simulink model "SetpointTransitionHandler"  (R2016b)
settings: Solver=FixedStepAuto  StartTime=0.0  StopTime=10.0  RelTol=1e-3  EnableMultiTasking=on
settings Model: Creator=march  LastModifiedBy=march
settings SolverCC: EnableConcurrentExecution=on
settings DataIOCC: SaveFormat=StructureWithTime
settings OptimizationCC: BlockReduction=off  OptimizeBlockIOStorage=off  BufferReuse=off  GlobalBufferReuse=off  ExpressionFolding=off  LocalBlockOutputs=off
settings HardwareCC: ProdBitPerPointer=32  ProdBitPerSizeT=32  ProdBitPerPtrDiffT=32  ProdLargestAtomicFloat=None  ProdWordSize=32  ProdLongLongMode=on  ProdHWDeviceType=Generic->32-bit x86 compatible
settings RTWCC: SystemTargetFile=slrt.tlc  TemplateMakefile=slrt_default_tmf  Description=Simulink Real-Time  RTWCompilerOptimization=on

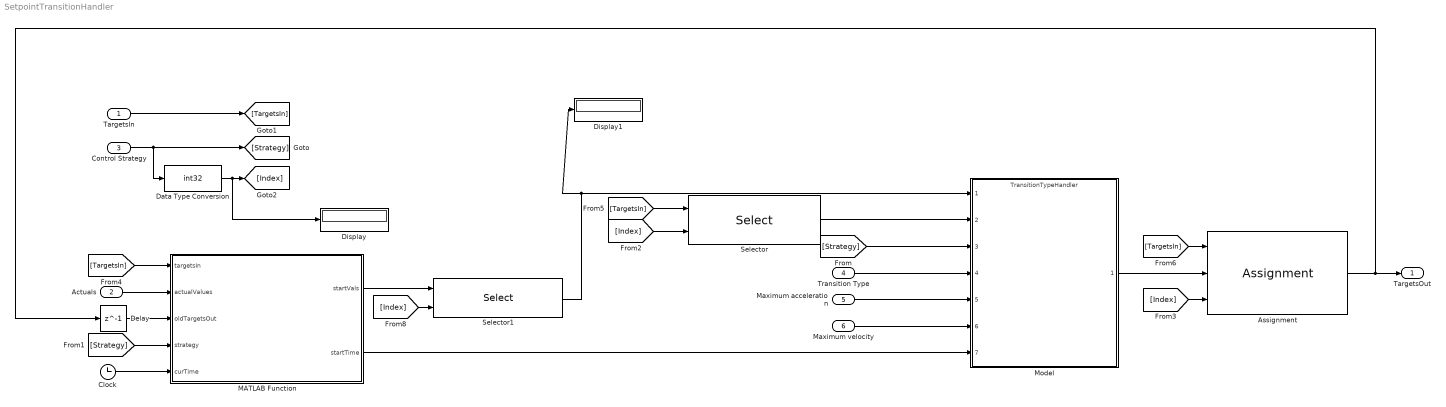
== system SetpointTransitionHandler ==
  TargetsIn : Inport  PortDimensions=[ 3 1 ]
  Actuals : Inport  Port=2  PortDimensions=[ 3 1 ]
  Control Strategy : Inport  Port=3  OutDataTypeStr=Enum: ControlStrategy
  Transition Type : Inport  Port=4
  Maximum acceleration : Inport  Port=5
  Maximum velocity : Inport  Port=6
  Assignment : Assignment  DiagnosticForDimensions=Warning  IndexOptions=Index vector (port)  Indices=1  OutputSizes=1
  Clock : Clock
  Data Type Conversion : DataTypeConversion  OutDataTypeStr=int32
  Delay : Delay  DelayLength=1
  Display : Display
  Display1 : Display
  MATLAB Function : MATLAB Function  TreatAsAtomicUnit=on
  Model : ModelReference  ModelNameDialog=TransitionTypeHandler  SimulationMode=Normal  ModelReferenceVersion=1.17
  Selector : Selector  InputPortWidth=3  IndexOptions=Index vector (port)  Indices=[1 3]  OutputSizes=1
  Selector1 : Selector  InputPortWidth=3  IndexOptions=Index vector (port)  Indices=[1 3]  OutputSizes=1
  TargetsOut : Outport
  wires:
  Delay/1 -> MATLAB Function/3(oldTargetsOut)
  Actuals/1 -> MATLAB Function/2(actualValues)
  Clock/1 -> MATLAB Function/5(curTime)
  Selector/1 -> Model/2
  MATLAB Function/2(startTime) -> Model/7
  MATLAB Function/1(startVals) -> Selector1/1
  Transition Type/1 -> Model/4
  Maximum acceleration/1 -> Model/5
  Maximum velocity/1 -> Model/6
  Model/1 -> Assignment/2
  Assignment/1 -> Delay/1, TargetsOut/1
  Control Strategy/1 -> [Strategy], Data Type Conversion/1
  [Strategy] -> Model/3
  [Strategy] -> MATLAB Function/4(strategy)
  [Index] -> Selector1/2
  [Index] -> Selector/2
  TargetsIn/1 -> [TargetsIn]
  [TargetsIn] -> MATLAB Function/1(targetsIn)
  [TargetsIn] -> Selector/1
  [TargetsIn] -> Assignment/1
  [Index] -> Assignment/3
  Data Type Conversion/1 -> Display/1, [Index]
  Selector1/1 -> Display1/1, Model/1

== matlab function SetpointTransitionHandler/MATLAB Function ==
  data: targetsIn input; actualValues input; startVals output; oldTargetsOut input; strategy input; curTime input; startTime output
function [startVals, startTime] = getStartValues( targetsIn, actualValues, oldTargetsOut, strategy, curTime)
persistent oldStart;
persistent prevTime;
persistent oldTargets;
persistent oldStrat;
if isempty(oldStart)
    oldStart = actualValues;
    oldTargets = targetsIn;
    prevTime = curTime;
    oldStrat = strategy;
end
closeEnough = 0.5;
hasReached = abs(targetsIn - oldTargetsOut) < closeEnough;
types = [ ControlStrategy.position; ControlStrategy.velocity; ControlStrategy.position ];
% The start value of the transition should be the actualValue of the 
% targetstrategy when changing strategies. When the targetOut has reached
% this targetIn, the actualValue should again be the startValue. For the
% types which arent the target strategy, always use actualValue as
% startValue
oldStart = or(types ~= strategy, hasReached).*actualValues + ...
    and(types == strategy, not(hasReached)).*oldStart;
startVals = oldStart;
if or(any(oldTargets ~= targetsIn), oldStrat ~= strategy)
    startTime = curTime;
else
    startTime = prevTime;
end
oldTargets = targetsIn;
oldStrat = strategy;
prevTime = startTime;
end
